simulink model "control_pos_6dof_conMI"  (R2023b)
settings: Solver=ode45  StartTime=0.0  StopTime=tsim  FixedStep=tstep  MaxStep=tstep
undefined symbols (not defined in the file): a0, a1, MI_Contr1, MI_Contr2, MI_Contr3, MI_Contr4, MI_Contr5, MI_Contr6, MI_motor1, MI_motor2, MI_motor3, MI_motor4, MI_motor5, MI_motor6, robot_params, sigbuilder_block, t_qeq_init, t_tr_init, tau_L, tr_ref
(part 4 of 10)

== system control_pos_6dof_conMI/Actuadores (Motores de inducción)/MI6 + PBC Torque Controller/Controlador PBC/Ley de control ==
  i_Sref : Inport
  d_iSref : Inport  Port=2
  psi_Rref : Inport  Port=3
  w_R : Inport  Port=4
  e_iS : Inport  Port=5
  Bus Selector : BusSelector  OutputSignals=epsilon_KiS
  K_iS : MATLAB Function  TreatAsAtomicUnit=on
  Ley de control : MATLAB Function  TreatAsAtomicUnit=on
  Scope17 : Scope
  U_S : Outport
  wires:
  [K_iS] -> Ley de control/7(KI_s)
  d_iSref/1 -> Ley de control/3(d_iSref)
  psi_Rref/1 -> Ley de control/4(psi_Rref)
  i_Sref/1 -> Ley de control/2(i_Sref)
  Ley de control/1(U_S) -> U_S/1
  w_R/1 -> [w_R], Ley de control/5(w_R)
  e_iS/1 -> Ley de control/6(e_Is)
  Bus Selector/1 -> K_iS/3(epsilon)  "<epsilon_KiS>"
  K_iS/1(K_iS) -> Scope17/1, [K_iS]
  [w_R] -> K_iS/2(w_R)
  [MI_motor_params] -> Ley de control/1(MI_motor_params)
  [MI_motor_params] -> K_iS/1(MI_motor_params)
  [PBC_params] -> Bus Selector/1

== system control_pos_6dof_conMI/Actuadores (Motores de inducción)/MI6 + PBC Torque Controller/Controlador PBC/Rampa+Ret ==
  Demux : Demux  Tag=STV Demux  Outputs=1
      settings: DisplayOption=none
  FromWs : FromWorkspace  Tag=STV FromWs  VariableName=tuvar
      SigBuilderData=|
      | common.afterFinalStr = 'Extrapolate'
      | common.sampleTime = 0
      | dataSet.timeRange = [0 20]
      | dataSet.name = 'Group 1'
      | sbobj.Groups.Name = 'Group 1'
      | sbobj.Groups.Signals.Name = 'Signal 1'
      | sbobj.Groups.Signals.XData = [0 0.5 1 20]
      | sbobj.Groups.Signals.YData = [0 0 0.64 0.64]
      | sbobj.Groups.TimeRange = [0 20]
  Signal 1 : Outport  Tag=STV Outport
  wires:
  Demux/1 -> Signal 1/1
  FromWs/1 -> Demux/1

== system control_pos_6dof_conMI/Actuadores (Motores de inducción)/MI6 + PBC Torque Controller/Controlador PBC/derivada Corrientes deseadas ==
  psi_Rref : Inport
  dpsi_Rref : Inport  Port=2
  psi_Rmagref : Inport  Port=3
  dpsi_Rmagref : Inport  Port=4
  ddpsi_Rmagref : Inport  Port=5
  tau_Rref : Inport  Port=6
  dtau_Rref : Inport  Port=7
  Scope10 : Scope
  derivada Corrientes deseadas : MATLAB Function  TreatAsAtomicUnit=on
  d_iSref : Outport
  wires:
  dpsi_Rref/1 -> derivada Corrientes deseadas/3(dpsi_Rref)
  tau_Rref/1 -> derivada Corrientes deseadas/7(tau_Rref)
  dtau_Rref/1 -> derivada Corrientes deseadas/8(dtau_Rref)
  dpsi_Rmagref/1 -> derivada Corrientes deseadas/5(dpsi_Rmagref)
  derivada Corrientes deseadas/1(d_iSref) -> Scope10/1, d_iSref/1
  psi_Rmagref/1 -> derivada Corrientes deseadas/4(psi_Rmagref)
  psi_Rref/1 -> derivada Corrientes deseadas/2(psi_Rref)
  ddpsi_Rmagref/1 -> derivada Corrientes deseadas/6(ddpsi_Rmagref)
  [MI_motor_params] -> derivada Corrientes deseadas/1(MI_motor_params)

== matlab function control_pos_6dof_conMI/Inicializar posición de robot manipulador/q_init/init_q3/Polinomio 7mo orden q0 ==
  data: t input; q0 input; qpol output; vpol output; apol output; jpol output; q1 input; t0 input; t1 input
function [qpol,vpol,apol,jpol] = fcn(t,q0,q1,t0,t1)


% t,q0,q1,v0,v1,ac0,ac1,j0,j1,t0,t1)
%Trayectoria de referencia

% q0 = 0;
% q1 = 0;

v0 = 0;
v1 = 0;

ac0 = 0;
ac1 = 0;

j0 = 0;
j1 = 0;

% t0 = 0;
% t1 = pi/4;

% Coeficientes de un polinomio de 7mo grado

h = q1 - q0;
T = t1 - t0;

a = zeros(7+1,1);

a(1) = q0;
a(2) = v0;
a(3) = ac0/2;
a(4) = j0/6;
a(5) = (210*h-T*((30*ac0-15*ac1)*T+(4*j0+j1)*T^2+120*v0+90*v1))/(6*T^4);
a(6) = (-168*h-T*((20*ac0-14*ac1)*T+(2*j0+j1)*T^2+90*v0+78*v1))/(2*T^5);
a(7) = (420*h-T*((45*ac0-39*ac1)*T+(4*j0+3*j1)*T^2+216*v0+204*v1))/(6*T^6);
a(8) = (-120*h-T*((12*ac0-12*ac1)*T+(j0+j1)*T^2+60*v0+60*v1))/(6*T^7);

qa = flip(a')';
va = polyder(qa')';
aa = polyder(va')';
ja = polyder(aa')';


if t>=t0 && t<t1
    qpol = polyval(qa,t-t0);
    vpol = polyval(va,t-t0);
    apol = polyval(aa,t-t0);
    jpol = polyval(ja,t-t0);
elseif t>=t1
    qpol = polyval(qa,T);
    vpol = polyval(va,T);
    apol = polyval(aa,T);
    jpol = polyval(ja,T);
else
    qpol = q0;
    vpol = v0;
    apol = ac0;
    jpol = j0;
end

== matlab function control_pos_6dof_conMI/Inicializar posición de robot manipulador/q_init/init_q3/Polinomio 7mo orden q1 ==
  data: t input; q0 input; qpol output; vpol output; apol output; jpol output; q1 input; t0 input; t1 input
function [qpol,vpol,apol,jpol] = fcn(t,q0,q1,t0,t1)


% t,q0,q1,v0,v1,ac0,ac1,j0,j1,t0,t1)
%Trayectoria de referencia

% q0 = 0;
% q1 = 0;

v0 = 0;
v1 = 0;

ac0 = 0;
ac1 = 0;

j0 = 0;
j1 = 0;

% t0 = 0;
% t1 = pi/4;

% Coeficientes de un polinomio de 7mo grado

h = q1 - q0;
T = t1 - t0;

a = zeros(7+1,1);

a(1) = q0;
a(2) = v0;
a(3) = ac0/2;
a(4) = j0/6;
a(5) = (210*h-T*((30*ac0-15*ac1)*T+(4*j0+j1)*T^2+120*v0+90*v1))/(6*T^4);
a(6) = (-168*h-T*((20*ac0-14*ac1)*T+(2*j0+j1)*T^2+90*v0+78*v1))/(2*T^5);
a(7) = (420*h-T*((45*ac0-39*ac1)*T+(4*j0+3*j1)*T^2+216*v0+204*v1))/(6*T^6);
a(8) = (-120*h-T*((12*ac0-12*ac1)*T+(j0+j1)*T^2+60*v0+60*v1))/(6*T^7);

qa = flip(a')';
va = polyder(qa')';
aa = polyder(va')';
ja = polyder(aa')';


if t>=t0 && t<t1
    qpol = polyval(qa,t-t0);
    vpol = polyval(va,t-t0);
    apol = polyval(aa,t-t0);
    jpol = polyval(ja,t-t0);
elseif t>=t1
    qpol = polyval(qa,T);
    vpol = polyval(va,T);
    apol = polyval(aa,T);
    jpol = polyval(ja,T);
else
    qpol = 0;
    vpol = 0;
    apol = 0;
    jpol = 0;
end

== matlab function control_pos_6dof_conMI/Inicializar posición de robot manipulador/q_init/init_q4/Polinomio 7mo orden q0 ==
  data: t input; q0 input; qpol output; vpol output; apol output; jpol output; q1 input; t0 input; t1 input
function [qpol,vpol,apol,jpol] = fcn(t,q0,q1,t0,t1)


% t,q0,q1,v0,v1,ac0,ac1,j0,j1,t0,t1)
%Trayectoria de referencia

% q0 = 0;
% q1 = 0;

v0 = 0;
v1 = 0;

ac0 = 0;
ac1 = 0;

j0 = 0;
j1 = 0;

% t0 = 0;
% t1 = pi/4;

% Coeficientes de un polinomio de 7mo grado

h = q1 - q0;
T = t1 - t0;

a = zeros(7+1,1);

a(1) = q0;
a(2) = v0;
a(3) = ac0/2;
a(4) = j0/6;
a(5) = (210*h-T*((30*ac0-15*ac1)*T+(4*j0+j1)*T^2+120*v0+90*v1))/(6*T^4);
a(6) = (-168*h-T*((20*ac0-14*ac1)*T+(2*j0+j1)*T^2+90*v0+78*v1))/(2*T^5);
a(7) = (420*h-T*((45*ac0-39*ac1)*T+(4*j0+3*j1)*T^2+216*v0+204*v1))/(6*T^6);
a(8) = (-120*h-T*((12*ac0-12*ac1)*T+(j0+j1)*T^2+60*v0+60*v1))/(6*T^7);

qa = flip(a')';
va = polyder(qa')';
aa = polyder(va')';
ja = polyder(aa')';


if t>=t0 && t<t1
    qpol = polyval(qa,t-t0);
    vpol = polyval(va,t-t0);
    apol = polyval(aa,t-t0);
    jpol = polyval(ja,t-t0);
elseif t>=t1
    qpol = polyval(qa,T);
    vpol = polyval(va,T);
    apol = polyval(aa,T);
    jpol = polyval(ja,T);
else
    qpol = q0;
    vpol = v0;
    apol = ac0;
    jpol = j0;
end

== matlab function control_pos_6dof_conMI/Inicializar posición de robot manipulador/q_init/init_q4/Polinomio 7mo orden q1 ==
  data: t input; q0 input; qpol output; vpol output; apol output; jpol output; q1 input; t0 input; t1 input
function [qpol,vpol,apol,jpol] = fcn(t,q0,q1,t0,t1)


% t,q0,q1,v0,v1,ac0,ac1,j0,j1,t0,t1)
%Trayectoria de referencia

% q0 = 0;
% q1 = 0;

v0 = 0;
v1 = 0;

ac0 = 0;
ac1 = 0;

j0 = 0;
j1 = 0;

% t0 = 0;
% t1 = pi/4;

% Coeficientes de un polinomio de 7mo grado

h = q1 - q0;
T = t1 - t0;

a = zeros(7+1,1);

a(1) = q0;
a(2) = v0;
a(3) = ac0/2;
a(4) = j0/6;
a(5) = (210*h-T*((30*ac0-15*ac1)*T+(4*j0+j1)*T^2+120*v0+90*v1))/(6*T^4);
a(6) = (-168*h-T*((20*ac0-14*ac1)*T+(2*j0+j1)*T^2+90*v0+78*v1))/(2*T^5);
a(7) = (420*h-T*((45*ac0-39*ac1)*T+(4*j0+3*j1)*T^2+216*v0+204*v1))/(6*T^6);
a(8) = (-120*h-T*((12*ac0-12*ac1)*T+(j0+j1)*T^2+60*v0+60*v1))/(6*T^7);

qa = flip(a')';
va = polyder(qa')';
aa = polyder(va')';
ja = polyder(aa')';


if t>=t0 && t<t1
    qpol = polyval(qa,t-t0);
    vpol = polyval(va,t-t0);
    apol = polyval(aa,t-t0);
    jpol = polyval(ja,t-t0);
elseif t>=t1
    qpol = polyval(qa,T);
    vpol = polyval(va,T);
    apol = polyval(aa,T);
    jpol = polyval(ja,T);
else
    qpol = 0;
    vpol = 0;
    apol = 0;
    jpol = 0;
end

== matlab function control_pos_6dof_conMI/Inicializar posición de robot manipulador/q_init/init_q5/Polinomio 7mo orden q0 ==
  data: t input; q0 input; qpol output; vpol output; apol output; jpol output; q1 input; t0 input; t1 input
function [qpol,vpol,apol,jpol] = fcn(t,q0,q1,t0,t1)


% t,q0,q1,v0,v1,ac0,ac1,j0,j1,t0,t1)
%Trayectoria de referencia

% q0 = 0;
% q1 = 0;

v0 = 0;
v1 = 0;

ac0 = 0;
ac1 = 0;

j0 = 0;
j1 = 0;

% t0 = 0;
% t1 = pi/4;

% Coeficientes de un polinomio de 7mo grado

h = q1 - q0;
T = t1 - t0;

a = zeros(7+1,1);

a(1) = q0;
a(2) = v0;
a(3) = ac0/2;
a(4) = j0/6;
a(5) = (210*h-T*((30*ac0-15*ac1)*T+(4*j0+j1)*T^2+120*v0+90*v1))/(6*T^4);
a(6) = (-168*h-T*((20*ac0-14*ac1)*T+(2*j0+j1)*T^2+90*v0+78*v1))/(2*T^5);
a(7) = (420*h-T*((45*ac0-39*ac1)*T+(4*j0+3*j1)*T^2+216*v0+204*v1))/(6*T^6);
a(8) = (-120*h-T*((12*ac0-12*ac1)*T+(j0+j1)*T^2+60*v0+60*v1))/(6*T^7);

qa = flip(a')';
va = polyder(qa')';
aa = polyder(va')';
ja = polyder(aa')';


if t>=t0 && t<t1
    qpol = polyval(qa,t-t0);
    vpol = polyval(va,t-t0);
    apol = polyval(aa,t-t0);
    jpol = polyval(ja,t-t0);
elseif t>=t1
    qpol = polyval(qa,T);
    vpol = polyval(va,T);
    apol = polyval(aa,T);
    jpol = polyval(ja,T);
else
    qpol = q0;
    vpol = v0;
    apol = ac0;
    jpol = j0;
end

== matlab function control_pos_6dof_conMI/Inicializar posición de robot manipulador/q_init/init_q5/Polinomio 7mo orden q1 ==
  data: t input; q0 input; qpol output; vpol output; apol output; jpol output; q1 input; t0 input; t1 input
function [qpol,vpol,apol,jpol] = fcn(t,q0,q1,t0,t1)


% t,q0,q1,v0,v1,ac0,ac1,j0,j1,t0,t1)
%Trayectoria de referencia

% q0 = 0;
% q1 = 0;

v0 = 0;
v1 = 0;

ac0 = 0;
ac1 = 0;

j0 = 0;
j1 = 0;

% t0 = 0;
% t1 = pi/4;

% Coeficientes de un polinomio de 7mo grado

h = q1 - q0;
T = t1 - t0;

a = zeros(7+1,1);

a(1) = q0;
a(2) = v0;
a(3) = ac0/2;
a(4) = j0/6;
a(5) = (210*h-T*((30*ac0-15*ac1)*T+(4*j0+j1)*T^2+120*v0+90*v1))/(6*T^4);
a(6) = (-168*h-T*((20*ac0-14*ac1)*T+(2*j0+j1)*T^2+90*v0+78*v1))/(2*T^5);
a(7) = (420*h-T*((45*ac0-39*ac1)*T+(4*j0+3*j1)*T^2+216*v0+204*v1))/(6*T^6);
a(8) = (-120*h-T*((12*ac0-12*ac1)*T+(j0+j1)*T^2+60*v0+60*v1))/(6*T^7);

qa = flip(a')';
va = polyder(qa')';
aa = polyder(va')';
ja = polyder(aa')';


if t>=t0 && t<t1
    qpol = polyval(qa,t-t0);
    vpol = polyval(va,t-t0);
    apol = polyval(aa,t-t0);
    jpol = polyval(ja,t-t0);
elseif t>=t1
    qpol = polyval(qa,T);
    vpol = polyval(va,T);
    apol = polyval(aa,T);
    jpol = polyval(ja,T);
else
    qpol = 0;
    vpol = 0;
    apol = 0;
    jpol = 0;
end

== matlab function control_pos_6dof_conMI/Inicializar posición de robot manipulador/q_init/init_q6/Polinomio 7mo orden q0 ==
  data: t input; q0 input; qpol output; vpol output; apol output; jpol output; q1 input; t0 input; t1 input
function [qpol,vpol,apol,jpol] = fcn(t,q0,q1,t0,t1)


% t,q0,q1,v0,v1,ac0,ac1,j0,j1,t0,t1)
%Trayectoria de referencia

% q0 = 0;
% q1 = 0;

v0 = 0;
v1 = 0;

ac0 = 0;
ac1 = 0;

j0 = 0;
j1 = 0;

% t0 = 0;
% t1 = pi/4;

% Coeficientes de un polinomio de 7mo grado

h = q1 - q0;
T = t1 - t0;

a = zeros(7+1,1);

a(1) = q0;
a(2) = v0;
a(3) = ac0/2;
a(4) = j0/6;
a(5) = (210*h-T*((30*ac0-15*ac1)*T+(4*j0+j1)*T^2+120*v0+90*v1))/(6*T^4);
a(6) = (-168*h-T*((20*ac0-14*ac1)*T+(2*j0+j1)*T^2+90*v0+78*v1))/(2*T^5);
a(7) = (420*h-T*((45*ac0-39*ac1)*T+(4*j0+3*j1)*T^2+216*v0+204*v1))/(6*T^6);
a(8) = (-120*h-T*((12*ac0-12*ac1)*T+(j0+j1)*T^2+60*v0+60*v1))/(6*T^7);

qa = flip(a')';
va = polyder(qa')';
aa = polyder(va')';
ja = polyder(aa')';


if t>=t0 && t<t1
    qpol = polyval(qa,t-t0);
    vpol = polyval(va,t-t0);
    apol = polyval(aa,t-t0);
    jpol = polyval(ja,t-t0);
elseif t>=t1
    qpol = polyval(qa,T);
    vpol = polyval(va,T);
    apol = polyval(aa,T);
    jpol = polyval(ja,T);
else
    qpol = q0;
    vpol = v0;
    apol = ac0;
    jpol = j0;
end

== matlab function control_pos_6dof_conMI/Inicializar posición de robot manipulador/q_init/init_q6/Polinomio 7mo orden q1 ==
  data: t input; q0 input; qpol output; vpol output; apol output; jpol output; q1 input; t0 input; t1 input
function [qpol,vpol,apol,jpol] = fcn(t,q0,q1,t0,t1)


% t,q0,q1,v0,v1,ac0,ac1,j0,j1,t0,t1)
%Trayectoria de referencia

% q0 = 0;
% q1 = 0;

v0 = 0;
v1 = 0;

ac0 = 0;
ac1 = 0;

j0 = 0;
j1 = 0;

% t0 = 0;
% t1 = pi/4;

% Coeficientes de un polinomio de 7mo grado

h = q1 - q0;
T = t1 - t0;

a = zeros(7+1,1);

a(1) = q0;
a(2) = v0;
a(3) = ac0/2;
a(4) = j0/6;
a(5) = (210*h-T*((30*ac0-15*ac1)*T+(4*j0+j1)*T^2+120*v0+90*v1))/(6*T^4);
a(6) = (-168*h-T*((20*ac0-14*ac1)*T+(2*j0+j1)*T^2+90*v0+78*v1))/(2*T^5);
a(7) = (420*h-T*((45*ac0-39*ac1)*T+(4*j0+3*j1)*T^2+216*v0+204*v1))/(6*T^6);
a(8) = (-120*h-T*((12*ac0-12*ac1)*T+(j0+j1)*T^2+60*v0+60*v1))/(6*T^7);

qa = flip(a')';
va = polyder(qa')';
aa = polyder(va')';
ja = polyder(aa')';


if t>=t0 && t<t1
    qpol = polyval(qa,t-t0);
    vpol = polyval(va,t-t0);
    apol = polyval(aa,t-t0);
    jpol = polyval(ja,t-t0);
elseif t>=t1
    qpol = polyval(qa,T);
    vpol = polyval(va,T);
    apol = polyval(aa,T);
    jpol = polyval(ja,T);
else
    qpol = 0;
    vpol = 0;
    apol = 0;
    jpol = 0;
end

== matlab function control_pos_6dof_conMI/q to xyz (robot)/Cinemática directa ==
  data: robot_params input; p output; q input
function p = fcn(robot_params,q)

l1 = robot_params.l(1);
l2 = robot_params.l(2);
l3 = robot_params.l(3);
l4 = robot_params.l(4);
l5 = robot_params.l(5);
l6 = robot_params.l(6);

d1 = robot_params.d(1);
d2 = robot_params.d(2);
d3 = robot_params.d(3);
d4 = robot_params.d(4);
d5 = robot_params.d(5);
d6 = robot_params.d(6);

q1 = q(1);
q2 = q(2);
q3 = q(3);
q4 = q(4);
q5 = q(5);
q6 = q(6);

% Cinematica directa %%%%%%%%%%%%%%%%%%%%%%%%%%%%%%%%%%%%%%%%%%%%%%%%%%%%%%

DH = [0   pi/2  d1 q1;
      l2  0     0  q2;
      l3  0     0  q3;
      0   pi/2  d4 q4;
      0   -pi/2 d5 q5;
      0   0     d6 q6];

A01 = transformacion_homogenea(DH(1,:));
A12 = transformacion_homogenea(DH(2,:));
A23 = transformacion_homogenea(DH(3,:));
A34 = transformacion_homogenea(DH(4,:));
A45 = transformacion_homogenea(DH(5,:));
A56 = transformacion_homogenea(DH(6,:));

T0 = zeros(4,4,6);

T0(:,:,1) = A01;
T0(:,:,2) = A01*A12;
T0(:,:,3) = A01*A12*A23;
T0(:,:,4) = A01*A12*A23*A34;
T0(:,:,5) = A01*A12*A23*A34*A45;
T0(:,:,6) = A01*A12*A23*A34*A45*A56;

p = reshape(T0(1:3,4,:),[3,6]);

end

function m = transformacion_homogenea(DH_i)
    a_i = DH_i(1);
    alpha_i = DH_i(2);
    d_i = DH_i(3);
    theta_i = DH_i(4);
    
    ma_i = [1 0 0 a_i;
            0 1 0 0;
            0 0 1 0;
            0 0 0 1];
    
    md_i = [1 0 0 0;
            0 1 0 0;
            0 0 1 d_i;
            0 0 0 1];
    
    mtheta_i = [cos(theta_i) -sin(theta_i) 0 0;
                sin(theta_i) cos(theta_i) 0 0;
                0 0 1 0;
                0 0 0 1];
    
    malpha_i = [1 0 0 0;
                0 cos(alpha_i) -sin(alpha_i) 0;
                0 sin(alpha_i) cos(alpha_i) 0;
                0 0 0 1];
    
    m = mtheta_i * md_i * ma_i * malpha_i;

end

== matlab function control_pos_6dof_conMI/Inicializar posición de robot manipulador/dq_init/q6/Polinomio 7mo orden dq ==
  data: t input; q0 input; qpol output; vpol output; apol output; jpol output; q1 input; t0 input; t1 input
function [qpol,vpol,apol,jpol] = fcn(t,q0,q1,t0,t1)


% t,q0,q1,v0,v1,ac0,ac1,j0,j1,t0,t1)
%Trayectoria de referencia

% q0 = 0;
% q1 = 0;

v0 = 0;
v1 = 0;

ac0 = 0;
ac1 = 0;

j0 = 0;
j1 = 0;

% t0 = 0;
% t1 = pi/4;

% Coeficientes de un polinomio de 7mo grado

h = q1 - q0;
T = t1 - t0;

a = zeros(7+1,1);

a(1) = q0;
a(2) = v0;
a(3) = ac0/2;
a(4) = j0/6;
a(5) = (210*h-T*((30*ac0-15*ac1)*T+(4*j0+j1)*T^2+120*v0+90*v1))/(6*T^4);
a(6) = (-168*h-T*((20*ac0-14*ac1)*T+(2*j0+j1)*T^2+90*v0+78*v1))/(2*T^5);
a(7) = (420*h-T*((45*ac0-39*ac1)*T+(4*j0+3*j1)*T^2+216*v0+204*v1))/(6*T^6);
a(8) = (-120*h-T*((12*ac0-12*ac1)*T+(j0+j1)*T^2+60*v0+60*v1))/(6*T^7);

qa = flip(a')';
va = polyder(qa')';
aa = polyder(va')';
ja = polyder(aa')';


if t>=t0 && t<t1
    qpol = polyval(qa,t-t0);
    vpol = polyval(va,t-t0);
    apol = polyval(aa,t-t0);
    jpol = polyval(ja,t-t0);
elseif t>=t1
    qpol = polyval(qa,T);
    vpol = polyval(va,T);
    apol = polyval(aa,T);
    jpol = polyval(ja,T);
else
    qpol = q0;
    vpol = v0;
    apol = ac0;
    jpol = j0;
end

== matlab function control_pos_6dof_conMI/Inicializar posición de robot manipulador/MATLAB Function ==
  data: t input size=1; qi output size=[6,1]; t_init input size=1; q input size=[6,1]; q_init input
function qi  = fcn(t,t_init,q,q_init)

% qi = q;
if t <= t_init
    qi = q;
else
    qi = q_init;
end

== matlab function control_pos_6dof_conMI/Inicializar posición de robot manipulador/dq_init1/q4/Polinomio 7mo orden dq ==
  data: t input; q0 input; qpol output; vpol output; apol output; jpol output; q1 input; t0 input; t1 input
function [qpol,vpol,apol,jpol] = fcn(t,q0,q1,t0,t1)


% t,q0,q1,v0,v1,ac0,ac1,j0,j1,t0,t1)
%Trayectoria de referencia

% q0 = 0;
% q1 = 0;

v0 = 0;
v1 = 0;

ac0 = 0;
ac1 = 0;

j0 = 0;
j1 = 0;

% t0 = 0;
% t1 = pi/4;

% Coeficientes de un polinomio de 7mo grado

h = q1 - q0;
T = t1 - t0;

a = zeros(7+1,1);

a(1) = q0;
a(2) = v0;
a(3) = ac0/2;
a(4) = j0/6;
a(5) = (210*h-T*((30*ac0-15*ac1)*T+(4*j0+j1)*T^2+120*v0+90*v1))/(6*T^4);
a(6) = (-168*h-T*((20*ac0-14*ac1)*T+(2*j0+j1)*T^2+90*v0+78*v1))/(2*T^5);
a(7) = (420*h-T*((45*ac0-39*ac1)*T+(4*j0+3*j1)*T^2+216*v0+204*v1))/(6*T^6);
a(8) = (-120*h-T*((12*ac0-12*ac1)*T+(j0+j1)*T^2+60*v0+60*v1))/(6*T^7);

qa = flip(a')';
va = polyder(qa')';
aa = polyder(va')';
ja = polyder(aa')';


if t>=t0 && t<t1
    qpol = polyval(qa,t-t0);
    vpol = polyval(va,t-t0);
    apol = polyval(aa,t-t0);
    jpol = polyval(ja,t-t0);
elseif t>=t1
    qpol = polyval(qa,T);
    vpol = polyval(va,T);
    apol = polyval(aa,T);
    jpol = polyval(ja,T);
else
    qpol = q0;
    vpol = v0;
    apol = ac0;
    jpol = j0;
end

== matlab function control_pos_6dof_conMI/Inicializar posición de robot manipulador/dq_init1/q5/Polinomio 7mo orden dq ==
  data: t input; q0 input; qpol output; vpol output; apol output; jpol output; q1 input; t0 input; t1 input
function [qpol,vpol,apol,jpol] = fcn(t,q0,q1,t0,t1)


% t,q0,q1,v0,v1,ac0,ac1,j0,j1,t0,t1)
%Trayectoria de referencia

% q0 = 0;
% q1 = 0;

v0 = 0;
v1 = 0;

ac0 = 0;
ac1 = 0;

j0 = 0;
j1 = 0;

% t0 = 0;
% t1 = pi/4;

% Coeficientes de un polinomio de 7mo grado

h = q1 - q0;
T = t1 - t0;

a = zeros(7+1,1);

a(1) = q0;
a(2) = v0;
a(3) = ac0/2;
a(4) = j0/6;
a(5) = (210*h-T*((30*ac0-15*ac1)*T+(4*j0+j1)*T^2+120*v0+90*v1))/(6*T^4);
a(6) = (-168*h-T*((20*ac0-14*ac1)*T+(2*j0+j1)*T^2+90*v0+78*v1))/(2*T^5);
a(7) = (420*h-T*((45*ac0-39*ac1)*T+(4*j0+3*j1)*T^2+216*v0+204*v1))/(6*T^6);
a(8) = (-120*h-T*((12*ac0-12*ac1)*T+(j0+j1)*T^2+60*v0+60*v1))/(6*T^7);

qa = flip(a')';
va = polyder(qa')';
aa = polyder(va')';
ja = polyder(aa')';


if t>=t0 && t<t1
    qpol = polyval(qa,t-t0);
    vpol = polyval(va,t-t0);
    apol = polyval(aa,t-t0);
    jpol = polyval(ja,t-t0);
elseif t>=t1
    qpol = polyval(qa,T);
    vpol = polyval(va,T);
    apol = polyval(aa,T);
    jpol = polyval(ja,T);
else
    qpol = q0;
    vpol = v0;
    apol = ac0;
    jpol = j0;
end

== matlab function control_pos_6dof_conMI/Inicializar posición de robot manipulador/dq_init1/q6/Polinomio 7mo orden dq ==
  data: t input; q0 input; qpol output; vpol output; apol output; jpol output; q1 input; t0 input; t1 input
function [qpol,vpol,apol,jpol] = fcn(t,q0,q1,t0,t1)


% t,q0,q1,v0,v1,ac0,ac1,j0,j1,t0,t1)
%Trayectoria de referencia

% q0 = 0;
% q1 = 0;

v0 = 0;
v1 = 0;

ac0 = 0;
ac1 = 0;

j0 = 0;
j1 = 0;

% t0 = 0;
% t1 = pi/4;

% Coeficientes de un polinomio de 7mo grado

h = q1 - q0;
T = t1 - t0;

a = zeros(7+1,1);

a(1) = q0;
a(2) = v0;
a(3) = ac0/2;
a(4) = j0/6;
a(5) = (210*h-T*((30*ac0-15*ac1)*T+(4*j0+j1)*T^2+120*v0+90*v1))/(6*T^4);
a(6) = (-168*h-T*((20*ac0-14*ac1)*T+(2*j0+j1)*T^2+90*v0+78*v1))/(2*T^5);
a(7) = (420*h-T*((45*ac0-39*ac1)*T+(4*j0+3*j1)*T^2+216*v0+204*v1))/(6*T^6);
a(8) = (-120*h-T*((12*ac0-12*ac1)*T+(j0+j1)*T^2+60*v0+60*v1))/(6*T^7);

qa = flip(a')';
va = polyder(qa')';
aa = polyder(va')';
ja = polyder(aa')';


if t>=t0 && t<t1
    qpol = polyval(qa,t-t0);
    vpol = polyval(va,t-t0);
    apol = polyval(aa,t-t0);
    jpol = polyval(ja,t-t0);
elseif t>=t1
    qpol = polyval(qa,T);
    vpol = polyval(va,T);
    apol = polyval(aa,T);
    jpol = polyval(ja,T);
else
    qpol = q0;
    vpol = v0;
    apol = ac0;
    jpol = j0;
end

== matlab function control_pos_6dof_conMI/Dinámica inversa (referencia)/Dinámica inversa ==
  data: robot_din input; dq input size=[6,1]; tau_s output size=[6,1]; ddq input size=[6,1]
function tau_s = fcn(robot_din,dq,ddq)

D = robot_din.D;
C = robot_din.C;
G = robot_din.G;
g = robot_din.g;

tau_s = D*ddq + C*dq + G*g;

== matlab function control_pos_6dof_conMI/Dinámica inversa (referencia)/Modelo dinámico ==
  data: robot_params input; robot_din output Bus: robot_din_bus size=1; q input size=[6,1]; dq input size=[6,1]
function robot_din = fcn(robot_params,q,dq)


% l1 = robot_params.l(1);
l2 = robot_params.l(2);
l3 = robot_params.l(3);
% l4 = robot_params.l(4);
% l5 = robot_params.l(5);
% l6 = robot_params.l(6);

lc1 = robot_params.lc(1);
lc2 = robot_params.lc(2);
lc3 = robot_params.lc(3);
% lc4 = robot_params.lc(4);
% lc5 = robot_params.lc(5);
% lc6 = robot_params.lc(6);

d1 = robot_params.d(1);
d2 = robot_params.d(2);
d3 = robot_params.d(3);
d4 = robot_params.d(4);
d5 = robot_params.d(5);
d6 = robot_params.d(6);

% dc1 = robot_params.dc(1);
% dc2 = robot_params.dc(2);
% dc3 = robot_params.dc(3);
dc4 = robot_params.dc(4);
dc5 = robot_params.dc(5);
dc6 = robot_params.dc(6);

m1 = robot_params.m(1);
m2 = robot_params.m(2);
m3 = robot_params.m(3);
m4 = robot_params.m(4);
m5 = robot_params.m(5);
m6 = robot_params.m(6);

%Posiciones angulares
% q1 = q(1);
q2 = q(2);
q3 = q(3);
q4 = q(4);
q5 = q(5);
% q6 = q(6);

%Velocidades angulares
dq1 = dq(1);
dq2 = dq(2);
dq3 = dq(3);
dq4 = dq(4);
dq5 = dq(5);
% dq6 = dq(6);

% Matriz de Inercia D
D = zeros(6,6);

D(1,1) = (d1*m1)/2 + (d2*m2)/2 + (d3*m3)/2 + (d4*m4)/2 + (d5*m5)/2 + (d6*m6)/2 + d4^2*m5 + d4^2*m6 + (d5^2*m6)/2 + dc4^2*m4 + (dc5^2*m5)/2 + (3*dc6^2*m6)/4 + (l2^2*m3)/2 + (l2^2*m4)/2 + (l2^2*m5)/2 + (l3^2*m4)/2 + (l2^2*m6)/2 + (l3^2*m5)/2 + (l3^2*m6)/2 + lc1^2*m1 + (lc2^2*m2)/2 + (lc3^2*m3)/2 - (dc6^2*m6*cos(2*q2 + 2*q3 + 2*q4 - 2*q5))/8 - (dc6^2*m6*cos(2*q2 + 2*q3 + 2*q4 + 2*q5))/8 - (d5^2*m6*cos(2*q2 + 2*q3 + 2*q4))/2 + (dc6^2*m6*cos(2*q5))/4 - (dc5^2*m5*cos(2*q2 + 2*q3 + 2*q4))/2 + (dc6^2*m6*cos(2*q2 + 2*q3 + 2*q4))/4 + (l2^2*m3*cos(2*q2))/2 + (l2^2*m4*cos(2*q2))/2 + (l2^2*m5*cos(2*q2))/2 + (l2^2*m6*cos(2*q2))/2 + (lc2^2*m2*cos(2*q2))/2 + (l3^2*m4*cos(2*q2 + 2*q3))/2 + (l3^2*m5*cos(2*q2 + 2*q3))/2 + (l3^2*m6*cos(2*q2 + 2*q3))/2 + (lc3^2*m3*cos(2*q2 + 2*q3))/2 + d5*l2*m6*sin(2*q2 + q3 + q4) + dc5*l2*m5*sin(2*q2 + q3 + q4) + (dc6*l2*m6*sin(q3 + q4 - q5))/2 + (d5*dc6*m6*cos(2*q2 + 2*q3 + 2*q4 + q5))/2 + d5*l2*m6*sin(q3 + q4) + dc5*l2*m5*sin(q3 + q4) - (dc6*l3*m6*sin(q4 + q5))/2 + (dc6*l3*m6*sin(2*q2 + 2*q3 + q4 - q5))/2 + 2*d4*dc6*m6*cos(q5) + l2*l3*m4*cos(q3) + l2*l3*m5*cos(q3) + l2*l3*m6*cos(q3) + l2*lc3*m3*cos(q3) + d5*l3*m6*sin(q4) + d5*l3*m6*sin(2*q2 + 2*q3 + q4) + dc5*l3*m5*sin(q4) + dc5*l3*m5*sin(2*q2 + 2*q3 + q4) - (dc6*l2*m6*sin(2*q2 + q3 + q4 + q5))/2 - (d5*dc6*m6*cos(2*q2 + 2*q3 + 2*q4 - q5))/2 + l2*l3*m4*cos(2*q2 + q3) + l2*l3*m5*cos(2*q2 + q3) + l2*l3*m6*cos(2*q2 + q3) + l2*lc3*m3*cos(2*q2 + q3) + (dc6*l3*m6*sin(q4 - q5))/2 - (dc6*l2*m6*sin(q3 + q4 + q5))/2 + (dc6*l2*m6*sin(2*q2 + q3 + q4 - q5))/2 - (dc6*l3*m6*sin(2*q2 + 2*q3 + q4 + q5))/2;
D(1,2) = (dc6^2*m6*cos(q2 + q3 + q4 - 2*q5))/4 - (dc6^2*m6*cos(q2 + q3 + q4 + 2*q5))/4 - (d4*dc6*m6*cos(q2 + q3 + q4 + q5))/2 + (d5*dc6*m6*cos(q2 + q3 + q4 + q5))/2 - (dc6*l3*m6*sin(q2 + q3 - q5))/2 - d4*l3*m5*sin(q2 + q3) - d4*l3*m6*sin(q2 + q3) - dc4*l3*m4*sin(q2 + q3) - (dc6*l2*m6*sin(q2 + q5))/2 + (d4*dc6*m6*cos(q2 + q3 + q4 - q5))/2 + (d5*dc6*m6*cos(q2 + q3 + q4 - q5))/2 - d4*l2*m5*sin(q2) - d4*l2*m6*sin(q2) - dc4*l2*m4*sin(q2) + d4*d5*m6*cos(q2 + q3 + q4) + d4*dc5*m5*cos(q2 + q3 + q4) - (dc6*l2*m6*sin(q2 - q5))/2 - (dc6*l3*m6*sin(q2 + q3 + q5))/2;
D(1,3) = (dc6^2*m6*cos(q2 + q3 + q4 - 2*q5))/4 - (dc6^2*m6*cos(q2 + q3 + q4 + 2*q5))/4 - (d4*dc6*m6*cos(q2 + q3 + q4 + q5))/2 + (d5*dc6*m6*cos(q2 + q3 + q4 + q5))/2 - (dc6*l3*m6*sin(q2 + q3 - q5))/2 - d4*l3*m5*sin(q2 + q3) - d4*l3*m6*sin(q2 + q3) - dc4*l3*m4*sin(q2 + q3) + (d4*dc6*m6*cos(q2 + q3 + q4 - q5))/2 + (d5*dc6*m6*cos(q2 + q3 + q4 - q5))/2 + d4*d5*m6*cos(q2 + q3 + q4) + d4*dc5*m5*cos(q2 + q3 + q4) - (dc6*l3*m6*sin(q2 + q3 + q5))/2;
D(1,4) = (dc6^2*m6*cos(q2 + q3 + q4 - 2*q5))/4 - (dc6^2*m6*cos(q2 + q3 + q4 + 2*q5))/4 - (d4*dc6*m6*cos(q2 + q3 + q4 + q5))/2 + (d5*dc6*m6*cos(q2 + q3 + q4 + q5))/2 + (d4*dc6*m6*cos(q2 + q3 + q4 - q5))/2 + (d5*dc6*m6*cos(q2 + q3 + q4 - q5))/2 + d4*d5*m6*cos(q2 + q3 + q4) + d4*dc5*m5*cos(q2 + q3 + q4);
D(1,5) = -(dc6*m6*(d4*cos(q2 + q3 + q4 + q5) + d5*cos(q2 + q3 + q4 + q5) + l3*sin(q2 + q3 - q5) - l2*sin(q2 + q5) + d4*cos(q2 + q3 + q4 - q5) - d5*cos(q2 + q3 + q4 - q5) + 2*dc6*cos(q2 + q3 + q4) + l2*sin(q2 - q5) - l3*sin(q2 + q3 + q5)))/2;
D(1,6) = 0;

D(2,1) = (dc6^2*m6*cos(q2 + q3 + q4 - 2*q5))/4 - (dc6^2*m6*cos(q2 + q3 + q4 + 2*q5))/4 - (d4*dc6*m6*cos(q2 + q3 + q4 + q5))/2 + (d5*dc6*m6*cos(q2 + q3 + q4 + q5))/2 - (dc6*l3*m6*sin(q2 + q3 - q5))/2 - d4*l3*m5*sin(q2 + q3) - d4*l3*m6*sin(q2 + q3) - dc4*l3*m4*sin(q2 + q3) - (dc6*l2*m6*sin(q2 + q5))/2 + (d4*dc6*m6*cos(q2 + q3 + q4 - q5))/2 + (d5*dc6*m6*cos(q2 + q3 + q4 - q5))/2 - d4*l2*m5*sin(q2) - d4*l2*m6*sin(q2) - dc4*l2*m4*sin(q2) + d4*d5*m6*cos(q2 + q3 + q4) + d4*dc5*m5*cos(q2 + q3 + q4) - (dc6*l2*m6*sin(q2 - q5))/2 - (dc6*l3*m6*sin(q2 + q3 + q5))/2;
D(2,2) = (d2*m2)/2 + (d3*m3)/2 + (d4*m4)/2 + (d5*m5)/2 + (d6*m6)/2 + d5^2*m6 + dc5^2*m5 + (dc6^2*m6)/2 + l2^2*m3 + l2^2*m4 + l2^2*m5 + l3^2*m4 + l2^2*m6 + l3^2*m5 + l3^2*m6 + lc2^2*m2 + lc3^2*m3 - (dc6^2*m6*cos(2*q5))/2 + 2*d5*l2*m6*sin(q3 + q4) + 2*dc5*l2*m5*sin(q3 + q4) + 2*l2*l3*m4*cos(q3) + 2*l2*l3*m5*cos(q3) + 2*l2*l3*m6*cos(q3) + 2*l2*lc3*m3*cos(q3) + 2*d5*l3*m6*sin(q4) + 2*dc5*l3*m5*sin(q4) - 2*dc6*l3*m6*cos(q4)*sin(q5) - 2*dc6*l2*m6*cos(q3)*cos(q4)*sin(q5) + 2*dc6*l2*m6*sin(q3)*sin(q4)*sin(q5);
D(2,3) = d5^2*m6 + dc5^2*m5 + (dc6^2*m6)/2 + l3^2*m4 + l3^2*m5 + l3^2*m6 + lc3^2*m3 - (dc6^2*m6*cos(2*q5))/2 + d5*l2*m6*sin(q3 + q4) + dc5*l2*m5*sin(q3 + q4) + l2*l3*m4*cos(q3) + l2*l3*m5*cos(q3) + l2*l3*m6*cos(q3) + l2*lc3*m3*cos(q3) + 2*d5*l3*m6*sin(q4) + 2*dc5*l3*m5*sin(q4) - 2*dc6*l3*m6*cos(q4)*sin(q5) - dc6*l2*m6*cos(q3)*cos(q4)*sin(q5) + dc6*l2*m6*sin(q3)*sin(q4)*sin(q5);
D(2,4) = d5^2*m6 + dc5^2*m5 + (dc6^2*m6)/2 - (dc6^2*m6*cos(2*q5))/2 + d5*l2*m6*sin(q3 + q4) + dc5*l2*m5*sin(q3 + q4) + d5*l3*m6*sin(q4) + dc5*l3*m5*sin(q4) - dc6*l3*m6*cos(q4)*sin(q5) - dc6*l2*m6*cos(q3)*cos(q4)*sin(q5) + dc6*l2*m6*sin(q3)*sin(q4)*sin(q5);
D(2,5) = -dc6*m6*cos(q5)*(d5 + l2*sin(q3 + q4) + l3*sin(q4));
D(2,6) = 0;

D(3,1) = (dc6^2*m6*cos(q2 + q3 + q4 - 2*q5))/4 - (dc6^2*m6*cos(q2 + q3 + q4 + 2*q5))/4 - (d4*dc6*m6*cos(q2 + q3 + q4 + q5))/2 + (d5*dc6*m6*cos(q2 + q3 + q4 + q5))/2 - (dc6*l3*m6*sin(q2 + q3 - q5))/2 - d4*l3*m5*sin(q2 + q3) - d4*l3*m6*sin(q2 + q3) - dc4*l3*m4*sin(q2 + q3) + (d4*dc6*m6*cos(q2 + q3 + q4 - q5))/2 + (d5*dc6*m6*cos(q2 + q3 + q4 - q5))/2 + d4*d5*m6*cos(q2 + q3 + q4) + d4*dc5*m5*cos(q2 + q3 + q4) - (dc6*l3*m6*sin(q2 + q3 + q5))/2;
D(3,2) = d5^2*m6 + dc5^2*m5 + (dc6^2*m6)/2 + l3^2*m4 + l3^2*m5 + l3^2*m6 + lc3^2*m3 - (dc6^2*m6*cos(2*q5))/2 + d5*l2*m6*sin(q3 + q4) + dc5*l2*m5*sin(q3 + q4) + l2*l3*m4*cos(q3) + l2*l3*m5*cos(q3) + l2*l3*m6*cos(q3) + l2*lc3*m3*cos(q3) + 2*d5*l3*m6*sin(q4) + 2*dc5*l3*m5*sin(q4) - 2*dc6*l3*m6*cos(q4)*sin(q5) - dc6*l2*m6*cos(q3)*cos(q4)*sin(q5) + dc6*l2*m6*sin(q3)*sin(q4)*sin(q5);
D(3,3) = (d3*m3)/2 + (d4*m4)/2 + (d5*m5)/2 + (d6*m6)/2 + d5^2*m6 + dc5^2*m5 + l3^2*m4 + l3^2*m5 + l3^2*m6 + lc3^2*m3 + dc6^2*m6*sin(q5)^2 + 2*d5*l3*m6*sin(q4) + 2*dc5*l3*m5*sin(q4) - 2*dc6*l3*m6*cos(q4)*sin(q5);
D(3,4) = d5^2*m6 + dc5^2*m5 + dc6^2*m6*sin(q5)^2 + d5*l3*m6*sin(q4) + dc5*l3*m5*sin(q4) - dc6*l3*m6*cos(q4)*sin(q5);
D(3,5) = -dc6*m6*cos(q5)*(d5 + l3*sin(q4));
D(3,6) = 0;

D(4,1) = (dc6^2*m6*cos(q2 + q3 + q4 - 2*q5))/4 - (dc6^2*m6*cos(q2 + q3 + q4 + 2*q5))/4 - (d4*dc6*m6*cos(q2 + q3 + q4 + q5))/2 + (d5*dc6*m6*cos(q2 + q3 + q4 + q5))/2 + (d4*dc6*m6*cos(q2 + q3 + q4 - q5))/2 + (d5*dc6*m6*cos(q2 + q3 + q4 - q5))/2 + d4*d5*m6*cos(q2 + q3 + q4) + d4*dc5*m5*cos(q2 + q3 + q4);
D(4,2) = d5^2*m6 + dc5^2*m5 + (dc6^2*m6)/2 - (dc6^2*m6*cos(2*q5))/2 + d5*l2*m6*sin(q3 + q4) + dc5*l2*m5*sin(q3 + q4) + d5*l3*m6*sin(q4) + dc5*l3*m5*sin(q4) - dc6*l3*m6*cos(q4)*sin(q5) - dc6*l2*m6*cos(q3)*cos(q4)*sin(q5) + dc6*l2*m6*sin(q3)*sin(q4)*sin(q5);
D(4,3) = d5^2*m6 + dc5^2*m5 + dc6^2*m6*sin(q5)^2 + d5*l3*m6*sin(q4) + dc5*l3*m5*sin(q4) - dc6*l3*m6*cos(q4)*sin(q5);
D(4,4) = (d4*m4)/2 + (d5*m5)/2 + (d6*m6)/2 + d5^2*m6 + dc5^2*m5 + dc6^2*m6 - dc6^2*m6*cos(q5)^2;
D(4,5) = -d5*dc6*m6*cos(q5);
D(4,6) = 0;

D(5,1) = -(dc6*m6*(d4*cos(q2 + q3 + q4 + q5) + d5*cos(q2 + q3 + q4 + q5) + l3*sin(q2 + q3 - q5) - l2*sin(q2 + q5) + d4*cos(q2 + q3 + q4 - q5) - d5*cos(q2 + q3 + q4 - q5) + 2*dc6*cos(q2 + q3 + q4) + l2*sin(q2 - q5) - l3*sin(q2 + q3 + q5)))/2;
D(5,2) = -dc6*m6*cos(q5)*(d5 + l2*sin(q3 + q4) + l3*sin(q4));
D(5,3) = -dc6*m6*cos(q5)*(d5 + l3*sin(q4));
D(5,4) = -d5*dc6*m6*cos(q5);
D(5,5) = (d5*m5)/2 + (d6*m6)/2 + dc6^2*m6;
D(5,6) = 0;

D(6,1) = 0;
D(6,2) = 0;
D(6,3) = 0;
D(6,4) = 0;
D(6,5) = 0;
D(6,6) = 1;

% Matriz de Coriollis C
C = zeros(6,6);

C(1,1) = 0;
C(1,2) = (dc6^2*dq1*m6*sin(2*q2 + 2*q3 + 2*q4 - 2*q5))/4 + (dc6^2*dq1*m6*sin(2*q2 + 2*q3 + 2*q4 + 2*q5))/4 + d5^2*dq1*m6*sin(2*q2 + 2*q3 + 2*q4) + dc5^2*dq1*m5*sin(2*q2 + 2*q3 + 2*q4) - (dc6^2*dq1*m6*sin(2*q2 + 2*q3 + 2*q4))/2 - dq1*l2^2*m3*sin(2*q2) - dq1*l2^2*m4*sin(2*q2) - dq1*l2^2*m5*sin(2*q2) - dq1*l2^2*m6*sin(2*q2) - dq1*lc2^2*m2*sin(2*q2) - dq1*l3^2*m4*sin(2*q2 + 2*q3) - dq1*l3^2*m5*sin(2*q2 + 2*q3) - dq1*l3^2*m6*sin(2*q2 + 2*q3) - dq1*lc3^2*m3*sin(2*q2 + 2*q3) - (dc6^2*dq2*m6*sin(q2 + q3 + q4 - 2*q5))/4 + (dc6^2*dq2*m6*sin(q2 + q3 + q4 + 2*q5))/4 - (dc6*dq2*l2*m6*cos(q2 - q5))/2 + d5*dc6*dq1*m6*sin(2*q2 + 2*q3 + 2*q4 - q5) - (dc6*dq2*l3*m6*cos(q2 + q3 + q5))/2 - 2*dq1*l2*l3*m4*sin(2*q2 + q3) - 2*dq1*l2*l3*m5*sin(2*q2 + q3) - 2*dq1*l2*l3*m6*sin(2*q2 + q3) - 2*dq1*l2*lc3*m3*sin(2*q2 + q3) - d4*d5*dq2*m6*sin(q2 + q3 + q4) - d4*dc5*dq2*m5*sin(q2 + q3 + q4) + dc6*dq1*l2*m6*cos(2*q2 + q3 + q4 - q5) - dc6*dq1*l3*m6*cos(2*q2 + 2*q3 + q4 + q5) + 2*d5*dq1*l2*m6*cos(2*q2 + q3 + q4) + 2*dc5*dq1*l2*m5*cos(2*q2 + q3 + q4) - (dc6*dq2*l3*m6*cos(q2 + q3 - q5))/2 + (d4*dc6*dq2*m6*sin(q2 + q3 + q4 + q5))/2 - (d5*dc6*dq2*m6*sin(q2 + q3 + q4 + q5))/2 - d4*dq2*l3*m5*cos(q2 + q3) - d4*dq2*l3*m6*cos(q2 + q3) - dc4*dq2*l3*m4*cos(q2 + q3) - (dc6*dq2*l2*m6*cos(q2 + q5))/2 + dc6*dq1*l3*m6*cos(2*q2 + 2*q3 + q4 - q5) - d5*dc6*dq1*m6*sin(2*q2 + 2*q3 + 2*q4 + q5) - d4*dq2*l2*m5*cos(q2) - d4*dq2*l2*m6*cos(q2) + 2*d5*dq1*l3*m6*cos(2*q2 + 2*q3 + q4) - dc4*dq2*l2*m4*cos(q2) + 2*dc5*dq1*l3*m5*cos(2*q2 + 2*q3 + q4) - dc6*dq1*l2*m6*cos(2*q2 + q3 + q4 + q5) - (d4*dc6*dq2*m6*sin(q2 + q3 + q4 - q5))/2 - (d5*dc6*dq2*m6*sin(q2 + q3 + q4 - q5))/2;
C(1,3) = (dc6^2*dq1*m6*sin(2*q2 + 2*q3 + 2*q4 - 2*q5))/4 + (dc6^2*dq1*m6*sin(2*q2 + 2*q3 + 2*q4 + 2*q5))/4 + d5^2*dq1*m6*sin(2*q2 + 2*q3 + 2*q4) + dc5^2*dq1*m5*sin(2*q2 + 2*q3 + 2*q4) - (dc6^2*dq1*m6*sin(2*q2 + 2*q3 + 2*q4))/2 - dq1*l3^2*m4*sin(2*q2 + 2*q3) - dq1*l3^2*m5*sin(2*q2 + 2*q3) - dq1*l3^2*m6*sin(2*q2 + 2*q3) - dq1*lc3^2*m3*sin(2*q2 + 2*q3) - (dc6^2*dq2*m6*sin(q2 + q3 + q4 - 2*q5))/2 + (dc6^2*dq2*m6*sin(q2 + q3 + q4 + 2*q5))/2 - (dc6^2*dq3*m6*sin(q2 + q3 + q4 - 2*q5))/4 + (dc6^2*dq3*m6*sin(q2 + q3 + q4 + 2*q5))/4 + d5*dc6*dq1*m6*sin(2*q2 + 2*q3 + 2*q4 - q5) - (dc6*dq1*l2*m6*cos(q3 + q4 + q5))/2 - dc6*dq2*l3*m6*cos(q2 + q3 + q5) - (dc6*dq3*l3*m6*cos(q2 + q3 + q5))/2 - dq1*l2*l3*m4*sin(2*q2 + q3) - dq1*l2*l3*m5*sin(2*q2 + q3) - dq1*l2*l3*m6*sin(2*q2 + q3) - dq1*l2*lc3*m3*sin(2*q2 + q3) - 2*d4*d5*dq2*m6*sin(q2 + q3 + q4) - d4*d5*dq3*m6*sin(q2 + q3 + q4) - 2*d4*dc5*dq2*m5*sin(q2 + q3 + q4) - d4*dc5*dq3*m5*sin(q2 + q3 + q4) + (dc6*dq1*l2*m6*cos(2*q2 + q3 + q4 - q5))/2 - dc6*dq1*l3*m6*cos(2*q2 + 2*q3 + q4 + q5) + d5*dq1*l2*m6*cos(2*q2 + q3 + q4) + dc5*dq1*l2*m5*cos(2*q2 + q3 + q4) + (dc6*dq1*l2*m6*cos(q3 + q4 - q5))/2 - dc6*dq2*l3*m6*cos(q2 + q3 - q5) - (dc6*dq3*l3*m6*cos(q2 + q3 - q5))/2 + d4*dc6*dq2*m6*sin(q2 + q3 + q4 + q5) + (d4*dc6*dq3*m6*sin(q2 + q3 + q4 + q5))/2 - d5*dc6*dq2*m6*sin(q2 + q3 + q4 + q5) - (d5*dc6*dq3*m6*sin(q2 + q3 + q4 + q5))/2 - 2*d4*dq2*l3*m5*cos(q2 + q3) - 2*d4*dq2*l3*m6*cos(q2 + q3) - d4*dq3*l3*m5*cos(q2 + q3) - d4*dq3*l3*m6*cos(q2 + q3) + d5*dq1*l2*m6*cos(q3 + q4) - 2*dc4*dq2*l3*m4*cos(q2 + q3) - dc4*dq3*l3*m4*cos(q2 + q3) + dc5*dq1*l2*m5*cos(q3 + q4) + dc6*dq1*l3*m6*cos(2*q2 + 2*q3 + q4 - q5) - d5*dc6*dq1*m6*sin(2*q2 + 2*q3 + 2*q4 + q5) + 2*d5*dq1*l3*m6*cos(2*q2 + 2*q3 + q4) + 2*dc5*dq1*l3*m5*cos(2*q2 + 2*q3 + q4) - (dc6*dq1*l2*m6*cos(2*q2 + q3 + q4 + q5))/2 - dq1*l2*l3*m4*sin(q3) - dq1*l2*l3*m5*sin(q3) - dq1*l2*l3*m6*sin(q3) - dq1*l2*lc3*m3*sin(q3) - d4*dc6*dq2*m6*sin(q2 + q3 + q4 - q5) - (d4*dc6*dq3*m6*sin(q2 + q3 + q4 - q5))/2 - d5*dc6*dq2*m6*sin(q2 + q3 + q4 - q5) - (d5*dc6*dq3*m6*sin(q2 + q3 + q4 - q5))/2;
C(1,4) = (dc6^2*dq1*m6*sin(2*q2 + 2*q3 + 2*q4 - 2*q5))/4 + (dc6^2*dq1*m6*sin(2*q2 + 2*q3 + 2*q4 + 2*q5))/4 + d5^2*dq1*m6*sin(2*q2 + 2*q3 + 2*q4) + dc5^2*dq1*m5*sin(2*q2 + 2*q3 + 2*q4) - (dc6^2*dq1*m6*sin(2*q2 + 2*q3 + 2*q4))/2 - (dc6^2*dq2*m6*sin(q2 + q3 + q4 - 2*q5))/2 + (dc6^2*dq2*m6*sin(q2 + q3 + q4 + 2*q5))/2 - (dc6^2*dq3*m6*sin(q2 + q3 + q4 - 2*q5))/2 + (dc6^2*dq3*m6*sin(q2 + q3 + q4 + 2*q5))/2 - (dc6^2*dq4*m6*sin(q2 + q3 + q4 - 2*q5))/4 + (dc6^2*dq4*m6*sin(q2 + q3 + q4 + 2*q5))/4 + (dc6*dq1*l3*m6*cos(q4 - q5))/2 + d5*dc6*dq1*m6*sin(2*q2 + 2*q3 + 2*q4 - q5) - (dc6*dq1*l2*m6*cos(q3 + q4 + q5))/2 - 2*d4*d5*dq2*m6*sin(q2 + q3 + q4) - 2*d4*d5*dq3*m6*sin(q2 + q3 + q4) - d4*d5*dq4*m6*sin(q2 + q3 + q4) - 2*d4*dc5*dq2*m5*sin(q2 + q3 + q4) - 2*d4*dc5*dq3*m5*sin(q2 + q3 + q4) - d4*dc5*dq4*m5*sin(q2 + q3 + q4) + (dc6*dq1*l2*m6*cos(2*q2 + q3 + q4 - q5))/2 - (dc6*dq1*l3*m6*cos(2*q2 + 2*q3 + q4 + q5))/2 + d5*dq1*l2*m6*cos(2*q2 + q3 + q4) + dc5*dq1*l2*m5*cos(2*q2 + q3 + q4) + (dc6*dq1*l2*m6*cos(q3 + q4 - q5))/2 + d4*dc6*dq2*m6*sin(q2 + q3 + q4 + q5) + d4*dc6*dq3*m6*sin(q2 + q3 + q4 + q5) - d5*dc6*dq2*m6*sin(q2 + q3 + q4 + q5) + (d4*dc6*dq4*m6*sin(q2 + q3 + q4 + q5))/2 - d5*dc6*dq3*m6*sin(q2 + q3 + q4 + q5) - (d5*dc6*dq4*m6*sin(q2 + q3 + q4 + q5))/2 + d5*dq1*l2*m6*cos(q3 + q4) + dc5*dq1*l2*m5*cos(q3 + q4) - (dc6*dq1*l3*m6*cos(q4 + q5))/2 + (dc6*dq1*l3*m6*cos(2*q2 + 2*q3 + q4 - q5))/2 - d5*dc6*dq1*m6*sin(2*q2 + 2*q3 + 2*q4 + q5) + d5*dq1*l3*m6*cos(q4) + d5*dq1*l3*m6*cos(2*q2 + 2*q3 + q4) + dc5*dq1*l3*m5*cos(q4) + dc5*dq1*l3*m5*cos(2*q2 + 2*q3 + q4) - (dc6*dq1*l2*m6*cos(2*q2 + q3 + q4 + q5))/2 - d4*dc6*dq2*m6*sin(q2 + q3 + q4 - q5) - d4*dc6*dq3*m6*sin(q2 + q3 + q4 - q5) - d5*dc6*dq2*m6*sin(q2 + q3 + q4 - q5) - (d4*dc6*dq4*m6*sin(q2 + q3 + q4 - q5))/2 - d5*dc6*dq3*m6*sin(q2 + q3 + q4 - q5) - (d5*dc6*dq4*m6*sin(q2 + q3 + q4 - q5))/2;
C(1,5) = (dc6*m6*(4*d4*dq2*sin(q2 + q3 + q4 - q5) - 2*dq1*l2*cos(2*q2 + q3 + q4 + q5) - 8*d4*dq1*sin(q5) + 4*d4*dq3*sin(q2 + q3 + q4 - q5) + 4*d4*dq4*sin(q2 + q3 + q4 - q5) - 2*d4*dq5*sin(q2 + q3 + q4 - q5) + 2*d5*dq5*sin(q2 + q3 + q4 - q5) + 2*dc6*dq2*sin(q2 + q3 + q4 - 2*q5) + 2*dc6*dq2*sin(q2 + q3 + q4 + 2*q5) + 2*dc6*dq3*sin(q2 + q3 + q4 - 2*q5) + 2*dc6*dq3*sin(q2 + q3 + q4 + 2*q5) + 2*dc6*dq4*sin(q2 + q3 + q4 - 2*q5) + 2*dc6*dq4*sin(q2 + q3 + q4 + 2*q5) - 2*dq1*l3*cos(q4 - q5) + 2*dq5*l2*cos(q2 - q5) - 2*d5*dq1*sin(2*q2 + 2*q3 + 2*q4 - q5) - dc6*dq1*sin(2*q2 + 2*q3 + 2*q4 - 2*q5) + dc6*dq1*sin(2*q2 + 2*q3 + 2*q4 + 2*q5) - 2*dq1*l2*cos(q3 + q4 + q5) + 2*dq5*l3*cos(q2 + q3 + q5) + 4*dc6*dq2*sin(q2 + q3 + q4) + 4*dc6*dq3*sin(q2 + q3 + q4) + 4*dc6*dq4*sin(q2 + q3 + q4) - 2*dc6*dq1*sin(2*q5) - 2*dq1*l2*cos(2*q2 + q3 + q4 - q5) - 2*dq1*l3*cos(2*q2 + 2*q3 + q4 + q5) - 2*dq1*l2*cos(q3 + q4 - q5) + 2*dq5*l3*cos(q2 + q3 - q5) + 4*d4*dq2*sin(q2 + q3 + q4 + q5) + 4*d4*dq3*sin(q2 + q3 + q4 + q5) + 4*d4*dq4*sin(q2 + q3 + q4 + q5) + 2*d4*dq5*sin(q2 + q3 + q4 + q5) + 2*d5*dq5*sin(q2 + q3 + q4 + q5) - 2*dq1*l3*cos(q4 + q5) + 2*dq5*l2*cos(q2 + q5) - 2*dq1*l3*cos(2*q2 + 2*q3 + q4 - q5) - 2*d5*dq1*sin(2*q2 + 2*q3 + 2*q4 + q5)))/4;
C(1,6) = 0;

C(2,1) = (dc6^2*dq1*m6*sin(2*q2 + 2*q3 + 2*q4))/4 - (dc6^2*dq1*m6*sin(2*q2 + 2*q3 + 2*q4 + 2*q5))/8 - (d5^2*dq1*m6*sin(2*q2 + 2*q3 + 2*q4))/2 - (dc5^2*dq1*m5*sin(2*q2 + 2*q3 + 2*q4))/2 - (dc6^2*dq1*m6*sin(2*q2 + 2*q3 + 2*q4 - 2*q5))/8 + (dq1*l2^2*m3*sin(2*q2))/2 + (dq1*l2^2*m4*sin(2*q2))/2 + (dq1*l2^2*m5*sin(2*q2))/2 + (dq1*l2^2*m6*sin(2*q2))/2 + (dq1*lc2^2*m2*sin(2*q2))/2 + (dq1*l3^2*m4*sin(2*q2 + 2*q3))/2 + (dq1*l3^2*m5*sin(2*q2 + 2*q3))/2 + (dq1*l3^2*m6*sin(2*q2 + 2*q3))/2 + (dq1*lc3^2*m3*sin(2*q2 + 2*q3))/2 - (d5*dc6*dq1*m6*sin(2*q2 + 2*q3 + 2*q4 - q5))/2 + dq1*l2*l3*m4*sin(2*q2 + q3) + dq1*l2*l3*m5*sin(2*q2 + q3) + dq1*l2*l3*m6*sin(2*q2 + q3) + dq1*l2*lc3*m3*sin(2*q2 + q3) - (dc6*dq1*l2*m6*cos(2*q2 + q3 + q4 - q5))/2 + (dc6*dq1*l3*m6*cos(2*q2 + 2*q3 + q4 + q5))/2 - d5*dq1*l2*m6*cos(2*q2 + q3 + q4) - dc5*dq1*l2*m5*cos(2*q2 + q3 + q4) - (dc6*dq1*l3*m6*cos(2*q2 + 2*q3 + q4 - q5))/2 + (d5*dc6*dq1*m6*sin(2*q2 + 2*q3 + 2*q4 + q5))/2 - d5*dq1*l3*m6*cos(2*q2 + 2*q3 + q4) - dc5*dq1*l3*m5*cos(2*q2 + 2*q3 + q4) + (dc6*dq1*l2*m6*cos(2*q2 + q3 + q4 + q5))/2;
C(2,2) = 0;
C(2,3) = -l2*(2*dq2 + dq3)*(l3*m4*sin(q3) + l3*m5*sin(q3) + l3*m6*sin(q3) + lc3*m3*sin(q3) - d5*m6*cos(q3 + q4) - dc5*m5*cos(q3 + q4) - dc6*m6*cos(q3)*sin(q4)*sin(q5) - dc6*m6*cos(q4)*sin(q3)*sin(q5));
C(2,4) = (dc6*dq4*l3*m6*cos(q4 - q5))/2 + 2*d5*dq2*l2*m6*cos(q3 + q4) + 2*d5*dq3*l2*m6*cos(q3 + q4) + d5*dq4*l2*m6*cos(q3 + q4) + 2*dc5*dq2*l2*m5*cos(q3 + q4) + 2*dc5*dq3*l2*m5*cos(q3 + q4) + dc5*dq4*l2*m5*cos(q3 + q4) - (dc6*dq4*l3*m6*cos(q4 + q5))/2 + 2*d5*dq2*l3*m6*cos(q4) + 2*d5*dq3*l3*m6*cos(q4) + d5*dq4*l3*m6*cos(q4) + 2*dc5*dq2*l3*m5*cos(q4) + 2*dc5*dq3*l3*m5*cos(q4) + dc5*dq4*l3*m5*cos(q4) + 2*dc6*dq2*l3*m6*sin(q4)*sin(q5) + 2*dc6*dq3*l3*m6*sin(q4)*sin(q5) + 2*dc6*dq2*l2*m6*cos(q3)*sin(q4)*sin(q5) + 2*dc6*dq2*l2*m6*cos(q4)*sin(q3)*sin(q5) + 2*dc6*dq3*l2*m6*cos(q3)*sin(q4)*sin(q5) + 2*dc6*dq3*l2*m6*cos(q4)*sin(q3)*sin(q5) + dc6*dq4*l2*m6*cos(q3)*sin(q4)*sin(q5) + dc6*dq4*l2*m6*cos(q4)*sin(q3)*sin(q5);
C(2,5) = -(dc6*m6*(2*dq2*l3*cos(q4 - q5) - 2*d5*dq1*sin(q2 + q3 + q4 - q5) - dc6*dq1*sin(q2 + q3 + q4 - 2*q5) - dc6*dq1*sin(q2 + q3 + q4 + 2*q5) - 2*dq1*l2*cos(q2 - q5) - 2*d5*dq5*sin(q5) + 2*dq3*l3*cos(q4 - q5) + 2*dq4*l3*cos(q4 - q5) - dq5*l3*cos(q4 - q5) + 2*dq1*l3*cos(q2 + q3 + q5) + 2*dq2*l2*cos(q3 + q4 + q5) + 2*dq3*l2*cos(q3 + q4 + q5) + 2*dq4*l2*cos(q3 + q4 + q5) + dq5*l2*cos(q3 + q4 + q5) + 2*dc6*dq1*sin(q2 + q3 + q4) - 2*dc6*dq2*sin(2*q5) - 2*dc6*dq3*sin(2*q5) - 2*dc6*dq4*sin(2*q5) - 2*dq1*l3*cos(q2 + q3 - q5) + 2*dq2*l2*cos(q3 + q4 - q5) + 2*dq3*l2*cos(q3 + q4 - q5) + 2*dq4*l2*cos(q3 + q4 - q5) - dq5*l2*cos(q3 + q4 - q5) + 2*d5*dq1*sin(q2 + q3 + q4 + q5) + 2*dq1*l2*cos(q2 + q5) + 2*dq2*l3*cos(q4 + q5) + 2*dq3*l3*cos(q4 + q5) + 2*dq4*l3*cos(q4 + q5) + dq5*l3*cos(q4 + q5)))/2;
C(2,6) = 0;

C(3,1) = (dc6^2*dq1*m6*sin(2*q2 + 2*q3 + 2*q4))/4 - (dc6^2*dq1*m6*sin(2*q2 + 2*q3 + 2*q4 + 2*q5))/8 - (d5^2*dq1*m6*sin(2*q2 + 2*q3 + 2*q4))/2 - (dc5^2*dq1*m5*sin(2*q2 + 2*q3 + 2*q4))/2 - (dc6^2*dq1*m6*sin(2*q2 + 2*q3 + 2*q4 - 2*q5))/8 + (dq1*l3^2*m4*sin(2*q2 + 2*q3))/2 + (dq1*l3^2*m5*sin(2*q2 + 2*q3))/2 + (dq1*l3^2*m6*sin(2*q2 + 2*q3))/2 + (dq1*lc3^2*m3*sin(2*q2 + 2*q3))/2 - (d5*dc6*dq1*m6*sin(2*q2 + 2*q3 + 2*q4 - q5))/2 + (dc6*dq1*l2*m6*cos(q3 + q4 + q5))/4 + (dq1*l2*l3*m4*sin(2*q2 + q3))/2 + (dq1*l2*l3*m5*sin(2*q2 + q3))/2 + (dq1*l2*l3*m6*sin(2*q2 + q3))/2 + (dq1*l2*lc3*m3*sin(2*q2 + q3))/2 - (dc6*dq1*l2*m6*cos(2*q2 + q3 + q4 - q5))/4 + (dc6*dq1*l3*m6*cos(2*q2 + 2*q3 + q4 + q5))/2 - (d5*dq1*l2*m6*cos(2*q2 + q3 + q4))/2 - (dc5*dq1*l2*m5*cos(2*q2 + q3 + q4))/2 - (dc6*dq1*l2*m6*cos(q3 + q4 - q5))/4 - (d5*dq1*l2*m6*cos(q3 + q4))/2 - (dc5*dq1*l2*m5*cos(q3 + q4))/2 - (dc6*dq1*l3*m6*cos(2*q2 + 2*q3 + q4 - q5))/2 + (d5*dc6*dq1*m6*sin(2*q2 + 2*q3 + 2*q4 + q5))/2 - d5*dq1*l3*m6*cos(2*q2 + 2*q3 + q4) - dc5*dq1*l3*m5*cos(2*q2 + 2*q3 + q4) + (dc6*dq1*l2*m6*cos(2*q2 + q3 + q4 + q5))/4 + (dq1*l2*l3*m4*sin(q3))/2 + (dq1*l2*l3*m5*sin(q3))/2 + (dq1*l2*l3*m6*sin(q3))/2 + (dq1*l2*lc3*m3*sin(q3))/2;
C(3,2) = dq2*l2*(l3*m4*sin(q3) + l3*m5*sin(q3) + l3*m6*sin(q3) + lc3*m3*sin(q3) - d5*m6*cos(q3 + q4) - dc5*m5*cos(q3 + q4) - dc6*m6*cos(q3)*sin(q4)*sin(q5) - dc6*m6*cos(q4)*sin(q3)*sin(q5));
C(3,3) = 0;
C(3,4) = l3*(2*dq2 + 2*dq3 + dq4)*(d5*m6*cos(q4) + dc5*m5*cos(q4) + dc6*m6*sin(q4)*sin(q5));
C(3,5) = -dc6*m6*(dq2*l3*cos(q4 - q5) - d5*dq1*sin(q2 + q3 + q4 - q5) - (dc6*dq1*sin(q2 + q3 + q4 - 2*q5))/2 - (dc6*dq1*sin(q2 + q3 + q4 + 2*q5))/2 - d5*dq5*sin(q5) + dq3*l3*cos(q4 - q5) + dq4*l3*cos(q4 - q5) - (dq5*l3*cos(q4 - q5))/2 + dq1*l3*cos(q2 + q3 + q5) + dc6*dq1*sin(q2 + q3 + q4) - dc6*dq2*sin(2*q5) - dc6*dq3*sin(2*q5) - dc6*dq4*sin(2*q5) - dq1*l3*cos(q2 + q3 - q5) + d5*dq1*sin(q2 + q3 + q4 + q5) + dq2*l3*cos(q4 + q5) + dq3*l3*cos(q4 + q5) + dq4*l3*cos(q4 + q5) + (dq5*l3*cos(q4 + q5))/2);
C(3,6) = 0;

C(4,1) = (dc6^2*dq1*m6*sin(2*q2 + 2*q3 + 2*q4))/4 - (dc6^2*dq1*m6*sin(2*q2 + 2*q3 + 2*q4 + 2*q5))/8 - (d5^2*dq1*m6*sin(2*q2 + 2*q3 + 2*q4))/2 - (dc5^2*dq1*m5*sin(2*q2 + 2*q3 + 2*q4))/2 - (dc6^2*dq1*m6*sin(2*q2 + 2*q3 + 2*q4 - 2*q5))/8 - (dc6*dq1*l3*m6*cos(q4 - q5))/4 - (d5*dc6*dq1*m6*sin(2*q2 + 2*q3 + 2*q4 - q5))/2 + (dc6*dq1*l2*m6*cos(q3 + q4 + q5))/4 - (dc6*dq1*l2*m6*cos(2*q2 + q3 + q4 - q5))/4 + (dc6*dq1*l3*m6*cos(2*q2 + 2*q3 + q4 + q5))/4 - (d5*dq1*l2*m6*cos(2*q2 + q3 + q4))/2 - (dc5*dq1*l2*m5*cos(2*q2 + q3 + q4))/2 - (dc6*dq1*l2*m6*cos(q3 + q4 - q5))/4 - (d5*dq1*l2*m6*cos(q3 + q4))/2 - (dc5*dq1*l2*m5*cos(q3 + q4))/2 + (dc6*dq1*l3*m6*cos(q4 + q5))/4 - (dc6*dq1*l3*m6*cos(2*q2 + 2*q3 + q4 - q5))/4 + (d5*dc6*dq1*m6*sin(2*q2 + 2*q3 + 2*q4 + q5))/2 - (d5*dq1*l3*m6*cos(q4))/2 - (d5*dq1*l3*m6*cos(2*q2 + 2*q3 + q4))/2 - (dc5*dq1*l3*m5*cos(q4))/2 - (dc5*dq1*l3*m5*cos(2*q2 + 2*q3 + q4))/2 + (dc6*dq1*l2*m6*cos(2*q2 + q3 + q4 + q5))/4;
C(4,2) = - dq2*(l2*cos(q3 + q4) + l3*cos(q4))*(d5*m6 + dc5*m5) - dc6*dq2*l3*m6*sin(q4)*sin(q5) - dc6*dq2*l2*m6*cos(q3)*sin(q4)*sin(q5) - dc6*dq2*l2*m6*cos(q4)*sin(q3)*sin(q5);
C(4,3) = -l3*(2*dq2 + dq3)*(d5*m6*cos(q4) + dc5*m5*cos(q4) + dc6*m6*sin(q4)*sin(q5));
C(4,4) = 0;
C(4,5) = (dc6*m6*(2*d5*dq5*sin(q5) + 2*d5*dq1*sin(q2 + q3 + q4 - q5) + dc6*dq1*sin(q2 + q3 + q4 - 2*q5) + dc6*dq1*sin(q2 + q3 + q4 + 2*q5) - 2*dc6*dq1*sin(q2 + q3 + q4) + 2*dc6*dq2*sin(2*q5) + 2*dc6*dq3*sin(2*q5) + 2*dc6*dq4*sin(2*q5) - 2*d5*dq1*sin(q2 + q3 + q4 + q5)))/2;
C(4,6) = 0;

C(5,1) = (dc6*dq1*m6*(2*dc6*sin(2*q5) + 2*l2*cos(2*q2 + q3 + q4 - q5) + 2*l3*cos(2*q2 + 2*q3 + q4 + q5) + 2*l2*cos(q3 + q4 - q5) + 2*l3*cos(q4 + q5) + 2*l3*cos(2*q2 + 2*q3 + q4 - q5) + 2*d5*sin(2*q2 + 2*q3 + 2*q4 + q5) + 8*d4*sin(q5) + 2*l2*cos(2*q2 + q3 + q4 + q5) + 2*l3*cos(q4 - q5) + 2*d5*sin(2*q2 + 2*q3 + 2*q4 - q5) + dc6*sin(2*q2 + 2*q3 + 2*q4 - 2*q5) - dc6*sin(2*q2 + 2*q3 + 2*q4 + 2*q5) + 2*l2*cos(q3 + q4 + q5)))/8;
C(5,2) = (dc6*m6*(dq2*l3*cos(q4 - q5) - dc6*dq1*sin(q2 + q3 + q4 - 2*q5) - dc6*dq1*sin(q2 + q3 + q4 + 2*q5) - 2*dq1*l2*cos(q2 - q5) - 2*d5*dq1*sin(q2 + q3 + q4 - q5) + 2*dq1*l3*cos(q2 + q3 + q5) + dq2*l2*cos(q3 + q4 + q5) + 2*dc6*dq1*sin(q2 + q3 + q4) - dc6*dq2*sin(2*q5) - 2*dq1*l3*cos(q2 + q3 - q5) + dq2*l2*cos(q3 + q4 - q5) + 2*d5*dq1*sin(q2 + q3 + q4 + q5) + 2*dq1*l2*cos(q2 + q5) + dq2*l3*cos(q4 + q5)))/2;
C(5,3) = (dc6*m6*(2*dq2*l3*cos(q4 - q5) - dc6*dq1*sin(q2 + q3 + q4 - 2*q5) - dc6*dq1*sin(q2 + q3 + q4 + 2*q5) - 2*d5*dq1*sin(q2 + q3 + q4 - q5) + dq3*l3*cos(q4 - q5) + 2*dq1*l3*cos(q2 + q3 + q5) + 2*dc6*dq1*sin(q2 + q3 + q4) - 2*dc6*dq2*sin(2*q5) - dc6*dq3*sin(2*q5) - 2*dq1*l3*cos(q2 + q3 - q5) + 2*d5*dq1*sin(q2 + q3 + q4 + q5) + 2*dq2*l3*cos(q4 + q5) + dq3*l3*cos(q4 + q5)))/2;
C(5,4) = -(dc6*m6*(2*d5*dq1*sin(q2 + q3 + q4 - q5) + dc6*dq1*sin(q2 + q3 + q4 - 2*q5) + dc6*dq1*sin(q2 + q3 + q4 + 2*q5) - 2*dc6*dq1*sin(q2 + q3 + q4) + 2*dc6*dq2*sin(2*q5) + 2*dc6*dq3*sin(2*q5) + dc6*dq4*sin(2*q5) - 2*d5*dq1*sin(q2 + q3 + q4 + q5)))/2;
C(5,5) = 0;
C(5,6) = 0;

C(6,1) = 0;
C(6,2) = 0;
C(6,3) = 0;
C(6,4) = 0;
C(6,5) = 0;
C(6,6) = 0;



% Matriz de Gravedad G: 
G = zeros(6,1);

G(1,1) = 0;

G(2,1) = l2*m3*cos(q2) + l2*m4*cos(q2) + l2*m5*cos(q2) + l2*m6*cos(q2) + lc2*m2*cos(q2) + (dc6*m6*sin(q2 + q3 + q4 - q5))/2 + d5*m6*sin(q2 + q3 + q4) + dc5*m5*sin(q2 + q3 + q4) - (dc6*m6*sin(q2 + q3 + q4 + q5))/2 + l3*m4*cos(q2 + q3) + l3*m5*cos(q2 + q3) + l3*m6*cos(q2 + q3) + lc3*m3*cos(q2 + q3);

G(3,1) = (dc6*m6*sin(q2 + q3 + q4 - q5))/2 + d5*m6*sin(q2 + q3 + q4) + dc5*m5*sin(q2 + q3 + q4) - (dc6*m6*sin(q2 + q3 + q4 + q5))/2 + l3*m4*cos(q2 + q3) + l3*m5*cos(q2 + q3) + l3*m6*cos(q2 + q3) + lc3*m3*cos(q2 + q3);

G(4,1) = (dc6*m6*sin(q2 + q3 + q4 - q5))/2 + d5*m6*sin(q2 + q3 + q4) + dc5*m5*sin(q2 + q3 + q4) - (dc6*m6*sin(q2 + q3 + q4 + q5))/2;

G(5,1) = -(dc6*m6*(sin(q2 + q3 + q4 + q5) + sin(q2 + q3 + q4 - q5)))/2;

G(6,1) = 0;

robot_din = struct('D',D,'C',C,'G',G,'g',9.81);

%busInfo = Simulink.Bus.createObject(robot_dyn);

== matlab function control_pos_6dof_conMI/xyz to q (referencia)/Cinemática inversa ==
  data: robot_params input; q output size=[6,1]; r input size=[3,1]; R input size=[3,3]
function q = fcn(robot_params,r,R)

%l1 = robot_params.l(1);
l2 = robot_params.l(2);
l3 = robot_params.l(3);
%l4 = robot_params.l(4);
%l5 = robot_params.l(5);
%l6 = robot_params.l(6);

d1 = robot_params.d(1);
%d2 = robot_params.d(2);
%d3 = robot_params.d(3);
d4 = robot_params.d(4);
d5 = robot_params.d(5);
d6 = robot_params.d(6);

Xr = r(1);
Yr = r(2);
Zr = r(3);

% Cinematica inversa %%%%%%%%%%%%%%%%%%%%%%%%%%%%%%%%%%%%%%%%%%%%%%%%%%%%%%

A = d6*R(2,3) - Yr;
B = Xr - d6*R(1,3);

q1 = - atan2(sqrt(B^2+A^2-d4^2),d4) + atan2(B,A); %signo

c1 = cos(q1);
s1 = sin(q1);

C = c1*R(1,1) + s1*R(2,1);
D = c1*R(2,2) - s1*R(1,2);
E = s1*R(1,1) - c1*R(2,1);

q5 = - atan2(sqrt(E^2+D^2),s1*R(1,3)-c1*R(2,3)); %signo

c5 = cos(q5);
s5 = sin(q5);

q6 = atan2(D/s5,E/s5);

c6 = cos(q6);
s6 = sin(q6);

F = c5*c6;  

q234 = atan2(R(3,1)*F-s6*C,F*C+s6*R(3,1));

c234 = cos(q234);
s234 = sin(q234);

KC = c1*Xr + s1*Yr - s234*d5 + c234*s5*d6;
KS = Zr - d1 + c234*d5 + s234*s5*d6;

c3 = (KS^2 + KC^2 - l2^2 - l3^2)/(2*l2*l3);
s3 = - sqrt(1-c3^2);

q3 = + atan2(s3,c3); %signo %no cambiar
q2 = atan2(KS,KC) - atan2(s3*l3,c3*l3+l2);
q4 = q234 - q2 - q3;


q = [q1;q2;q3;q4;q5;q6];

== matlab function control_pos_6dof_conMI/q to xyz (referencia)/Cinemática directa ==
  data: robot_params input; p output; q input
function p = fcn(robot_params,q)

l1 = robot_params.l(1);
l2 = robot_params.l(2);
l3 = robot_params.l(3);
l4 = robot_params.l(4);
l5 = robot_params.l(5);
l6 = robot_params.l(6);

d1 = robot_params.d(1);
d2 = robot_params.d(2);
d3 = robot_params.d(3);
d4 = robot_params.d(4);
d5 = robot_params.d(5);
d6 = robot_params.d(6);

q1 = q(1);
q2 = q(2);
q3 = q(3);
q4 = q(4);
q5 = q(5);
q6 = q(6);

% Cinematica directa %%%%%%%%%%%%%%%%%%%%%%%%%%%%%%%%%%%%%%%%%%%%%%%%%%%%%%

DH = [0   pi/2  d1 q1;
      l2  0     0  q2;
      l3  0     0  q3;
      0   pi/2  d4 q4;
      0   -pi/2 d5 q5;
      0   0     d6 q6];

A01 = transformacion_homogenea(DH(1,:));
A12 = transformacion_homogenea(DH(2,:));
A23 = transformacion_homogenea(DH(3,:));
A34 = transformacion_homogenea(DH(4,:));
A45 = transformacion_homogenea(DH(5,:));
A56 = transformacion_homogenea(DH(6,:));

T0 = zeros(4,4,6);

T0(:,:,1) = A01;
T0(:,:,2) = A01*A12;
T0(:,:,3) = A01*A12*A23;
T0(:,:,4) = A01*A12*A23*A34;
T0(:,:,5) = A01*A12*A23*A34*A45;
T0(:,:,6) = A01*A12*A23*A34*A45*A56;

p = reshape(T0(1:3,4,:),[3,6]);

end

function m = transformacion_homogenea(DH_i)
    a_i = DH_i(1);
    alpha_i = DH_i(2);
    d_i = DH_i(3);
    theta_i = DH_i(4);
    
    ma_i = [1 0 0 a_i;
            0 1 0 0;
            0 0 1 0;
            0 0 0 1];
    
    md_i = [1 0 0 0;
            0 1 0 0;
            0 0 1 d_i;
            0 0 0 1];
    
    mtheta_i = [cos(theta_i) -sin(theta_i) 0 0;
                sin(theta_i) cos(theta_i) 0 0;
                0 0 1 0;
                0 0 0 1];
    
    malpha_i = [1 0 0 0;
                0 cos(alpha_i) -sin(alpha_i) 0;
                0 sin(alpha_i) cos(alpha_i) 0;
                0 0 0 1];
    
    m = mtheta_i * md_i * ma_i * malpha_i;

end
